simulink model "PCS_average_12_4"  (R2024a)
settings: Solver=FixedStepAuto  StartTime=0.0  StopTime=30.0  RelTol=1e-3
undefined symbols (not defined in the file or in its folder): DiscIntNeverNeededParam, initial, Ion, Lithium
libraries: spsCurrentMeasurementLib x16, spsVoltageMeasurementLib x13, spsControlledVoltageSourceLib x7, spsSeriesRLCBranchLib x5, spsThreePhaseSeriesRLCBranchLib x5, spsGroundLib x2, spsControlledCurrentSourceLib x2, slpidlib x2, SimplusGT x2, spsBatteryLib x1, dspfdesign x1, sps_lib x1
(part 1 of 2)
settings Model: NumberOfSteps=10  Creator=liao  LastModifiedBy=liao

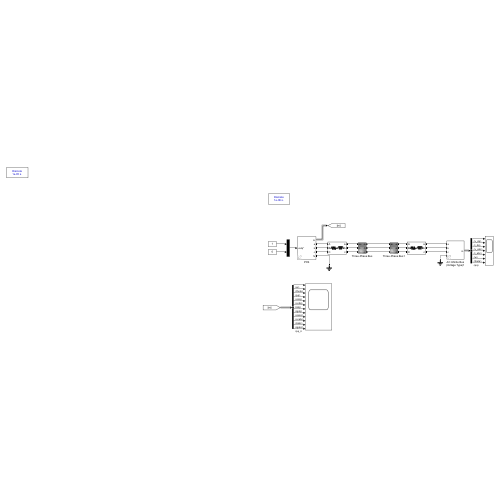
[thumbnail: Simulink's stored preview of the top-level diagram]
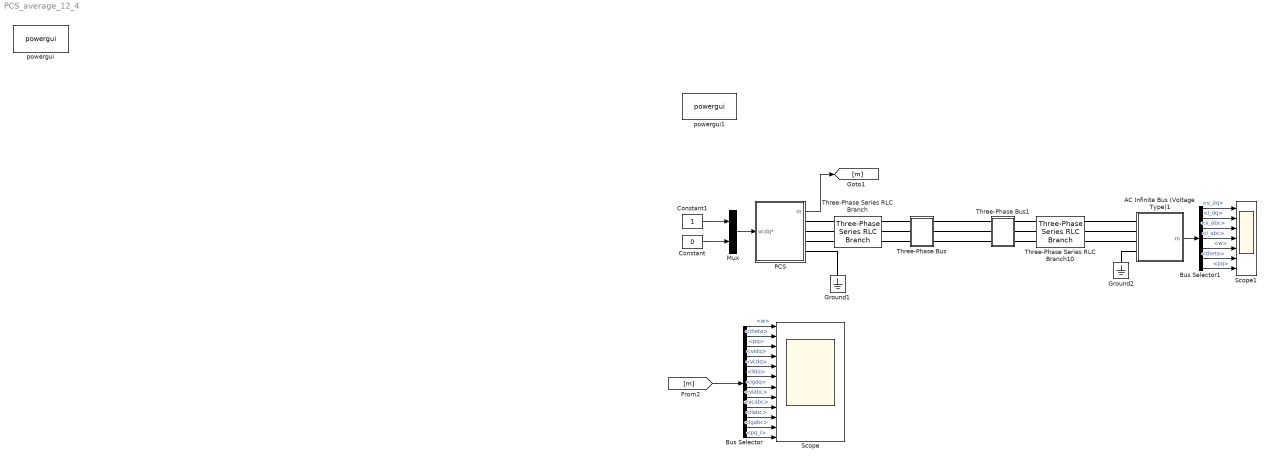
== system PCS_average_12_4 ==
  AC Infinite Bus (Voltage Type)1 : Subsystem  AncestorBlock=|  mask{Ts=1/10e3, Sbase=1, Vbase=1, Wbase=100*pi, vd=1, vq=0, theta0=0, w=100*pi, R=1e-30}
      | SimplusGT/AC Infinite Bus
      | (Voltage Type)
      mask prompts: Ts "Ts (s), samping period"; Sbase "Sbase (VA), power base"; Vbase "Vbase (V), voltage base"; Wbase "Wbase (rad/s), frequency base"; vd "vd (pu), d-axis voltage"; vq "vq (pu), q-axis voltage"; theta0 "theta0 (rad), initial angle"; w "w (rad/s), frequency"; R "R (Ohm), resistance"
      settings: LibrarySourceBlock=|
      | SimplusGT/AC Infinite Bus
      | (Voltage Type)
  Bus Selector : BusSelector  OutputSignals=w,theta,pq,vidq,vcdq,ildq,igdq,viabc,vcabc,ilabc,igabc,pq_i
  Bus Selector1 : BusSelector  OutputSignals=v_dq,i_dq,v_abc,i_abc,w,theta,pq
  Constant : Constant  Value=0
  Constant1 : Constant
  Ground1 : spsGroundLib/Ground  LConnTagsString=a
  Ground2 : spsGroundLib/Ground  LConnTagsString=a
  Mux : Mux  Inputs=2
  PCS : Subsystem  AncestorBlock=|  mask{Ts=1/10e3, Sbase=1, Vbase=1, Wbase=100*pi, w_i=1000*2*pi, w_v=250*2*pi, w_droop=10*2*pi, m=0.08, Lf=0.05, Cf=0.02, Lc=1e-30, Vbase_dc=1, Sbase_dc=1, L_dc=0.000125, C_dc=0.224, Bat_Cap=0.1, SOC_i=100}
      | SimplusGT/Grid-Forming Inverter
      | (Simulink Block)
      mask prompts: Ts "Ts (s), sampling period"; Sbase "Sbase (VA), base power"; Vbase "Vbase (V), base voltage"; Wbase "Wbase (rad/s), base frequency"; w_i "w_i (rad/s), current-loop bandwidth"; w_v "w_v (rad/s), voltage-loop bandwidth"; w_droop "w_droop (rad/s), droop bandwidth"; m "m (pu), frequency droop gain"; Lf "Lf (pu), LCL filter"; Cf "Cf (pu), LCL filter"; Lc "Lc (pu), LCL filter"; Vbase_dc "DC link base voltage"; Sbase_dc "DC link base power"; L_dc "DC link inductance(pu)"; C_dc "DC link super-capacitor(pu)"; Bat_Cap "Battery Capacity(Ah)"; SOC_i "Battery initial State of Charge(%)"
  Scope : Scope  NumInputPorts=12
  Scope1 : Scope  NumInputPorts=7
  Three-Phase Series RLC Branch : spsThreePhaseSeriesRLCBranchLib/Three-Phase Series RLC Branch  LConnTagsString=A|B|C  RConnTagsString=A|B|C  BranchType=RL  Resistance=0.25/5  Inductance=0.25/100/pi  Capacitance=1e-6  Measurements=None
  Three-Phase Series RLC Branch10 : spsThreePhaseSeriesRLCBranchLib/Three-Phase Series RLC Branch  LConnTagsString=A|B|C  RConnTagsString=A|B|C  BranchType=RL  Resistance=0.25/5  Inductance=0.25/100/pi  Capacitance=1e-6  Measurements=None
  Three-Phase Bus : Subsystem  AncestorBlock=SimplusGT/Three-Phase Bus  mask{Vbase=1, Sbase=1}
      settings: LibrarySourceBlock=SimplusGT/Three-Phase Bus
  Three-Phase Bus1 : Subsystem  AncestorBlock=SimplusGT/Three-Phase Bus  mask{Vbase=1, Sbase=1}
      settings: LibrarySourceBlock=SimplusGT/Three-Phase Bus
  powergui : sps_lib/powergui  Priority=1  SimulationMode=Discrete  SampleTime=0.00001  frequency=60  Iterations=50  frequencyindice=0  Pbase=100e6  ErrMax=1e-4  UnitsV=kV  UnitsW=MW  buscounter=0  FunctionMessages=off  echomessages=off  EnableUseOfTLC=off  CurrentSourceSwitches=off  DisableSnubberDevices=off  DisableRonSwitches=off  DisableVfSwitches=off  DisplayEquations=off  AutomaticDiscreteSolvers=off  SolverType=Tustin/Backward Euler (TBE)  Interpol=off  ExternalGateDelay=off  methode=off  Ts=100  x0status=blocks  SPID=on  SwTol=0  HookPort=off  NonlinearTolerance=1e-4  nMaxIteration=100  ContinueOnMaxIteration=off  RestoreLinks=warning  ResistiveCurrentMeasurement=off  Frange=[0:2:500]  Ylog=off  Xlog=on  ShowGrid=off  save=off  variable=ZData  structure=0  ZoomFFT=off  StartTime=0.0  cycles=1  DisplayStyle=1  fundamental=60  FreqAxis=off  MaxFrequency=1000  frequencyindicesteady=1  RmsSteady=1  display=off
  powergui1 : spspowerguiLib/powergui  Priority=1  SimulationMode=Discrete  SampleTime=0.000001  frequency=60  Iterations=50  frequencyindice=0  Pbase=100e6  ErrMax=1e-4  UnitsV=kV  UnitsW=MW  buscounter=0  FunctionMessages=off  echomessages=off  EnableUseOfTLC=off  CurrentSourceSwitches=off  DisableSnubberDevices=off  DisableRonSwitches=off  DisableVfSwitches=off  DisplayEquations=off  AutomaticDiscreteSolvers=off  SolverType=Tustin/Backward Euler (TBE)  Interpol=off  ExternalGateDelay=off  methode=off  Ts=100  x0status=blocks  SPID=on  SwTol=0  HookPort=off  NonlinearTolerance=1e-4  nMaxIteration=100  ContinueOnMaxIteration=off  RestoreLinks=warning  ResistiveCurrentMeasurement=off  Frange=[0:2:500]  Ylog=off  Xlog=on  ShowGrid=off  save=off  variable=ZData  structure=0  ZoomFFT=off  StartTime=0.0  cycles=1  DisplayStyle=1  fundamental=60  FreqAxis=off  MaxFrequency=1000  frequencyindicesteady=1  RmsSteady=1  display=off
  wires:
  Constant/1 -> Mux/2
  Mux/1 -> PCS/1(vcdq*)
  Constant1/1 -> Mux/1
  PCS/1(m) -> [m]
  Bus Selector1/5 -> Scope1/5  "<w>"
  Bus Selector1/1 -> Scope1/1  "<v_dq>"
  Bus Selector1/6 -> Scope1/6  "<theta>"
  Bus Selector1/4 -> Scope1/4  "<i_abc>"
  Bus Selector1/7 -> Scope1/7  "<pq>"
  Bus Selector1/3 -> Scope1/3  "<v_abc>"
  Bus Selector1/2 -> Scope1/2  "<i_dq>"
  AC Infinite Bus (Voltage Type)1/1(m) -> Bus Selector1/1
  [m] -> Bus Selector/1
  Bus Selector/1 -> Scope/1  "<w>"
  Bus Selector/2 -> Scope/2  "<theta>"
  Bus Selector/3 -> Scope/3  "<pq>"
  Bus Selector/4 -> Scope/4  "<vidq>"
  Bus Selector/5 -> Scope/5  "<vcdq>"
  Bus Selector/6 -> Scope/6  "<ildq>"
  Bus Selector/7 -> Scope/7  "<igdq>"
  Bus Selector/8 -> Scope/8  "<viabc>"
  Bus Selector/9 -> Scope/9  "<vcabc>"
  Bus Selector/10 -> Scope/10  "<ilabc>"
  Bus Selector/11 -> Scope/11  "<igabc>"
  Bus Selector/12 -> Scope/12  "<pq_i>"
  connections:
  Three-Phase Bus/RConn1 -- Three-Phase Bus1/LConn1
  Three-Phase Bus/RConn3 -- Three-Phase Bus1/LConn3
  Three-Phase Series RLC Branch10/RConn2 -- AC Infinite Bus (Voltage Type)1/LConn2
  Three-Phase Series RLC Branch10/RConn1 -- AC Infinite Bus (Voltage Type)1/LConn1
  Three-Phase Bus/LConn2 -- Three-Phase Series RLC Branch/RConn2
  Three-Phase Bus/LConn1 -- Three-Phase Series RLC Branch/RConn1
  Three-Phase Bus/LConn3 -- Three-Phase Series RLC Branch/RConn3
  PCS/RConn4 -- Ground1/LConn1
  PCS/RConn1 -- Three-Phase Series RLC Branch/LConn1
  Three-Phase Bus1/RConn2 -- Three-Phase Series RLC Branch10/LConn2
  Three-Phase Bus1/RConn3 -- Three-Phase Series RLC Branch10/LConn3
  Ground2/LConn1 -- AC Infinite Bus (Voltage Type)1/LConn4
  PCS/RConn2 -- Three-Phase Series RLC Branch/LConn2
  Three-Phase Bus1/RConn1 -- Three-Phase Series RLC Branch10/LConn1
  PCS/RConn3 -- Three-Phase Series RLC Branch/LConn3
  Three-Phase Series RLC Branch10/RConn3 -- AC Infinite Bus (Voltage Type)1/LConn3
  Three-Phase Bus/RConn2 -- Three-Phase Bus1/LConn2

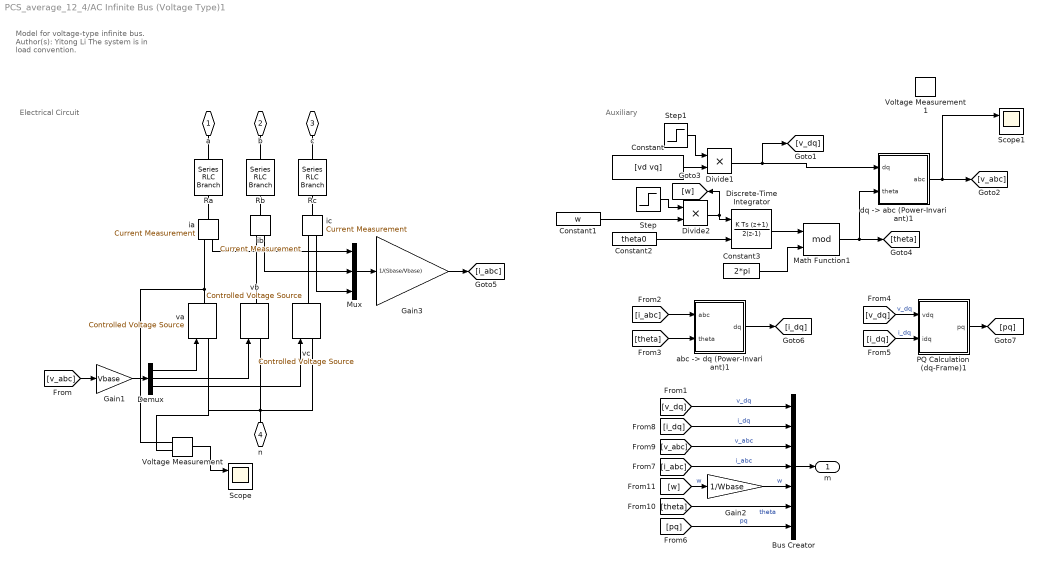
== system PCS_average_12_4/AC Infinite Bus (Voltage Type)1 ==
  note: Auxiliary
  note: Electrical Circuit
  note: Model for voltage-type infinite bus.
      |
      | Author(s): Yitong Li
      |
      | The system is in load convention.
  Bus Creator : BusCreator  Inputs=7
  Constant : Constant  Value=[vd vq]
  Constant1 : Constant  Value=w
  Constant2 : Constant  Value=theta0
  Constant3 : Constant  Value=2*pi
  Demux : Demux  Outputs=3
  Discrete-Time Integrator : DiscreteIntegrator  IntegratorMethod=Integration: Trapezoidal  InitialConditionSource=external  SampleTime=-1  ICPrevOutput=DiscIntNeverNeededParam  ICPrevScaledInput=DiscIntNeverNeededParam
  Divide1 : Product  Inputs=**
  Divide2 : Product  Inputs=**
  Gain1 : Gain  Gain=Vbase
  Gain2 : Gain  Gain=1/Wbase
  Gain3 : Gain  Gain=1/(Sbase/Vbase)
  Math Function1 : Math  Operator=mod  SignedPower=on
  Mux : Mux  Inputs=3
  PQ Calculation (dq-Frame)1 : Subsystem  AncestorBlock=|
      | SimplusGT/PQ Calculation
      | (dq-Frame)
      settings: LibrarySourceBlock=|
      | SimplusGT/PQ Calculation
      | (dq-Frame)
  Ra : spsSeriesRLCBranchLib/Series RLC Branch  LConnTagsString=__new0  RConnTagsString=__new0  BranchType=R  Resistance=R  Inductance=1e-3  SetiL0=off  InitialCurrent=0  Capacitance=1e-6  Setx0=off  InitialVoltage=0  Measurements=None
  Rb : spsSeriesRLCBranchLib/Series RLC Branch  LConnTagsString=__new0  RConnTagsString=__new0  BranchType=R  Resistance=R  Inductance=1e-3  SetiL0=off  InitialCurrent=0  Capacitance=1e-6  Setx0=off  InitialVoltage=0  Measurements=None
  Rc : spsSeriesRLCBranchLib/Series RLC Branch  LConnTagsString=__new0  RConnTagsString=__new0  BranchType=R  Resistance=R  Inductance=1e-3  SetiL0=off  InitialCurrent=0  Capacitance=1e-6  Setx0=off  InitialVoltage=0  Measurements=None
  Scope : Scope  NumInputPorts=2
  Scope1 : Scope  NumInputPorts=2
  Step : Step  Time=15  Before=0.9  After=1.1  SampleTime=0
  Step1 : Step  Time=0.5  Before=1  SampleTime=0
  Voltage Measurement : spsVoltageMeasurementLib/Voltage Measurement  PhasorSimulation=off  OutputType=Complex  PSBequivalent=0
  Voltage Measurement1 : spsVoltageMeasurementLib/Voltage Measurement  PhasorSimulation=off  OutputType=Complex  PSBequivalent=0
  "abc -> dq (Power-Invariant)1" : Subsystem  AncestorBlock=|
      | SimplusGT/abc -> dq
      | (Power-Invariant)
      settings: LibrarySourceBlock=|
      | SimplusGT/abc -> dq
      | (Power-Invariant)
  "dq -> abc (Power-Invariant)1" : Subsystem  AncestorBlock=|
      | SimplusGT/dq -> abc
      | (Power-Invariant)
      settings: LibrarySourceBlock=|
      | SimplusGT/dq -> abc
      | (Power-Invariant)
  ia : spsCurrentMeasurementLib/Current Measurement  PhasorSimulation=off  OutputType=Complex  PSBequivalent=0
  ib : spsCurrentMeasurementLib/Current Measurement  PhasorSimulation=off  OutputType=Complex  PSBequivalent=0
  ic : spsCurrentMeasurementLib/Current Measurement  PhasorSimulation=off  OutputType=Complex  PSBequivalent=0
  va : spsControlledVoltageSourceLib/Controlled Voltage Source  Initialize=on  Source_Type=AC  Amplitude=0  Phase=0  Frequency=0  Measurements=None
  vb : spsControlledVoltageSourceLib/Controlled Voltage Source  Initialize=on  Source_Type=AC  Amplitude=0  Phase=0  Frequency=0  Measurements=None
  vc : spsControlledVoltageSourceLib/Controlled Voltage Source  Initialize=on  Source_Type=AC  Amplitude=0  Phase=0  Frequency=0  Measurements=None
  a : PMIOPort  Side=Left
  b : PMIOPort  Port=2  Side=Left
  c : PMIOPort  Port=3  Side=Left
  n : PMIOPort  Port=4  Side=Left
  m : Outport
  wires:
  [pq] -> Bus Creator/7  "pq"
  PQ Calculation (dq-Frame)1/1(pq) -> [pq]
  [i_dq] -> PQ Calculation (dq-Frame)1/2(idq)  "i_dq"
  [v_dq] -> PQ Calculation (dq-Frame)1/1(vdq)  "v_dq"
  Gain3/1 -> [i_abc]
  Mux/1 -> Gain3/1
  Gain1/1 -> Demux/1
  "abc -> dq (Power-Invariant)1"/1(dq) -> [i_dq]
  [theta] -> "abc -> dq (Power-Invariant)1"/2(theta)
  [i_abc] -> "abc -> dq (Power-Invariant)1"/1(abc)
  ic/1 -> Mux/3
  ib/1 -> Mux/2
  ia/1 -> Mux/1
  [theta] -> Bus Creator/6  "theta"
  Bus Creator/1 -> m/1
  [i_dq] -> Bus Creator/2  "i_dq"
  Gain2/1 -> Bus Creator/5  "w"
  [v_abc] -> Bus Creator/3  "v_abc"
  [w] -> Gain2/1  "w"
  [i_abc] -> Bus Creator/4  "i_abc"
  [v_dq] -> Bus Creator/1  "v_dq"
  Discrete-Time Integrator/1 -> Math Function1/1
  Constant3/1 -> Math Function1/2
  "dq -> abc (Power-Invariant)1"/1(abc) -> Scope1/1, [v_abc]
  Constant1/1 -> Divide2/2
  Constant2/1 -> Discrete-Time Integrator/2
  Math Function1/1 -> [theta], "dq -> abc (Power-Invariant)1"/2(theta)
  Demux/3 -> vc/1
  Demux/2 -> vb/1
  Demux/1 -> va/1
  [v_abc] -> Gain1/1
  Voltage Measurement/1 -> Scope/1
  Step/1 -> Divide2/1
  Divide2/1 -> Discrete-Time Integrator/1, [w]
  Constant/1 -> Divide1/2
  Divide1/1 -> [v_dq], "dq -> abc (Power-Invariant)1"/1(dq)
  Step1/1 -> Divide1/1
  connections:
  Rc/LConn1 -- c/RConn1
  Rc/RConn1 -- ic/LConn1
  Rb/LConn1 -- b/RConn1
  ib/LConn1 -- Rb/RConn1
  Ra/LConn1 -- a/RConn1
  Ra/RConn1 -- ia/LConn1
  ic/RConn1 -- vc/RConn1
  ib/RConn1 -- vb/RConn1
  ia/RConn1 -- Voltage Measurement/LConn1 -- va/RConn1
  vb/LConn1 -- Voltage Measurement/LConn2 -- va/LConn1 -- n/RConn1 -- vc/LConn1

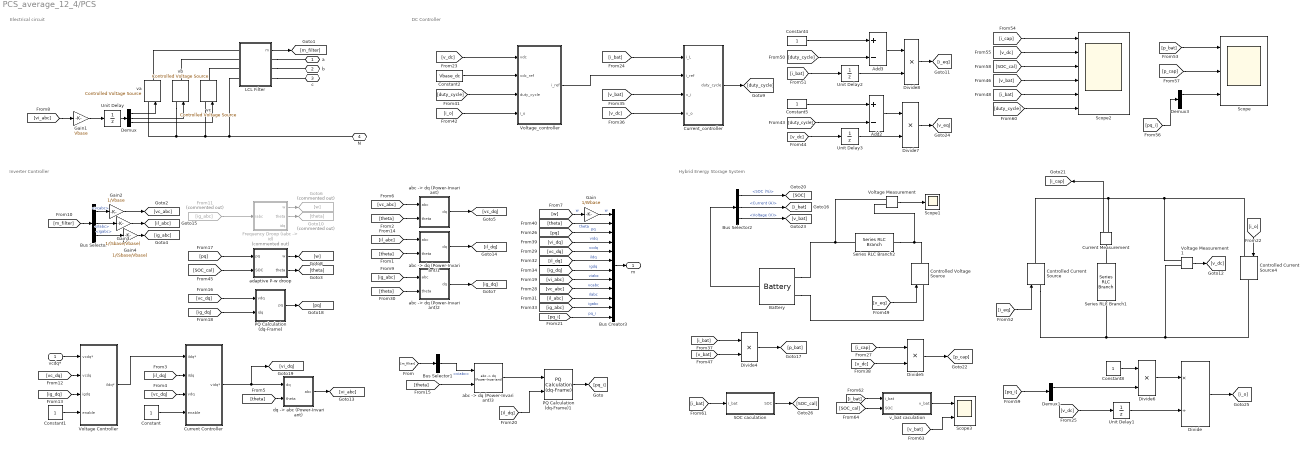
== system PCS_average_12_4/PCS ==
  note: Electrical circuit
  note: Inverter Controller
  note: Hybrid Energy Storage System
  note: DC Controller
  vcdq* : Inport
  Add2 : Sum  Inputs=+-
  Add3 : Sum  Inputs=+-
  Battery : spsBatteryLib/Battery  BatType=Lithium-Ion  ShowTempParam=off  ThermalPreset=no  ShowAgeParam=off  NomV=0.625*Vbase_dc  NomQ=Bat_Cap  SOC=SOC_i  Batt_Tr=30  PresetModel=on  MaxQ=0.1  MinV=0.46875  FullV=0.72749  Dis_rate=0.043478  R=0.0625  Normal_OP=0.090435  expZone="[0.67524    0.004913]"  current=[6.5 16 32.5]  Units=Time  Tci=20  NomT=20  T2=-30  MaxQ2=4.8  FullV2=7.1  Normal_OP2=5.655  expZone2="[6.58           1]"  Rca=0.6  ti=2000  Dp=0  Neq0=0  Tsim=1e6  Ta1=25  Qeol=5.4*0.9  Reol=0.013333*1.2  Char_age=[2.3478, 3]  Dis_age=[2.3478, 10]  N1=1500  N2=10500  N3=1000  N4=1400  Ta2=45  N5=950
  Bus Creator3 : BusCreator  Inputs=12
  Bus Selector : BusSelector  OutputSignals=vcabc,ilabc,igabc
  Bus Selector1 : BusSelector  OutputSignals=viabc
  Bus Selector2 : BusSelector  OutputSignals=SOC (%),Current (A),Voltage (V)
  Constant{,1,4..5,8} (5 alike) : Constant
  Constant2 : Constant  Value=Vbase_dc
  Controlled Current Source : spsControlledCurrentSourceLib/Controlled Current Source  Initialize=on  Source_Type=AC  Amplitude=0  Phase=0  Frequency=0  Measurements=None
  Controlled Current Source4 : spsControlledCurrentSourceLib/Controlled Current Source  Initialize=on  Source_Type=AC  Amplitude=0  Phase=0  Frequency=0  Measurements=None
  Controlled Voltage Source : spsControlledVoltageSourceLib/Controlled Voltage Source  Initialize=on  Source_Type=AC  Amplitude=0  Phase=0  Frequency=0  Measurements=None
  Current Controller : Subsystem  mask{Ts=Ts, Wbase=Wbase, Lf=Lf/Wbase, Kg=0, Kp=w_i*Lf/Wbase, Ki=w_i*w_i/4*Lf/Wbase, xdmax=inf, xqmax=inf, Kcd=0}
      mask prompts: Ts "Sampling Time (s)"; Wbase "Base Angular Frequency (rad/s)"; Lf "Inductance"; Kg "Estimator Gain"; Kp "Proportional Gain"; Ki "Integral Gain"; xdmax "Voltage D Limit"; xqmax "Voltage Q Limit"; Kcd "Cross Decoupling Gain"
  Current Measurement : spsCurrentMeasurementLib/Current Measurement  PhasorSimulation=off  OutputType=Complex  PSBequivalent=0
  Current_controller : Subsystem  mask{w_i=500*2*pi, L=L_dc*Sbase_dc/(Vbase_dc*Vbase_dc), flag_vi_decouple=0, flag_vo_decouple=1}
      mask prompts: w_i "current loop bandwidth"; L "L filter"; flag_vi_decouple "Input voltage decoupling flag"; flag_vo_decouple "Output voltage decoupling flag"
      mask DialogControl ParameterGroupVar Prompt: 参数
  Demux : Demux  Outputs=3
  Demux1 : Demux  Outputs=2
  Demux3 : Demux  Outputs=2
  Divide : Product  Inputs=*/
  Divide{4..8} (5 alike) : Product  Inputs=**
  "Frequency Droop (iabc -> id)" : Subsystem  Commented=on  AncestorBlock=|  mask{Ts=Ts, Sbase=Sbase, Vbase=Vbase, Wbase=Wbase, m=m, w_tau=w_droop, theta0=0, i0=0, w0=1}
      | SimplusGT/Frequency Droop
      | (iabc -> id)
      mask prompts: Ts "Ts (s), samping period"; Sbase "Sbase (VA), base power"; Vbase "Vbase (V), base voltage"; Wbase "Wbase (rad/s), base angular frequency"; m "m (pu), droop gain"; w_tau "w_tau (rad/s), low-pass filter bandwidth"; theta0 "theta0 (rad), initial angle"; i0 "i0 (pu), current setting point"; w0 "w0 (pu), frequency setting point"
  From11 : From  Commented=on  GotoTag=ig_abc
      settings: CloseFcn=tagdialog Close
  Gain : Gain  Gain=1/Wbase
  Gain1 : Gain  Gain=Vbase
  Gain2 : Gain  Gain=1/Vbase
  Gain3 : Gain  Gain=1/(Sbase/Vbase)
  Gain4 : Gain  Gain=1/(Sbase/Vbase)
  Goto10 : Goto  Commented=on  GotoTag=theta
  Goto6 : Goto  Commented=on  GotoTag=w
  LCL Filter : Subsystem  mask{Lf=Lf*(Vbase^2/Sbase)/Wbase, Rf=Lf*(Vbase^2/Sbase)/5, Lc=Lc*(Vbase^2/Sbase)/Wbase, Rc=Lc*(Vbase^2/Sbase)/5, Cf=Cf*(Sbase/Vbase^2)/Wbase, Rd=1e-5*(Vbase^2/Sbase)}
      mask prompts: Lf "Lf (H)"; Rf "Rf (Ohm)"; Lc "Lc (H)"; Rc "Rc (Ohm)"; Cf "Cf (F)"; Rd "Rd (Ohm)"
  PQ Calculation (dq-Frame) : Subsystem  AncestorBlock=|
      | SimplusGT/PQ Calculation
      | (dq-Frame)
  PQ Calculation (dq-Frame)1 : SimplusGT/PQ Calculation (dq-Frame)  SystemSampleTime=-1  VariantActivationTime=update diagram  AllowFlexibleInterface=on  Latency=0  AutoFrameSizeCalculation=off
      settings: SourceProductName=Simplus Grid Tool
  SOC caculation : Subsystem
  Scope : Scope  NumInputPorts=3
  Scope1 : Scope
  Scope2 : Scope  NumInputPorts=6
  Scope3 : Scope  NumInputPorts=2
  Series RLC Branch1 : spsSeriesRLCBranchLib/Series RLC Branch  LConnTagsString=__new0  RConnTagsString=__new0  BranchType=C  Resistance=1  Inductance=1e-3  SetiL0=off  InitialCurrent=0  Capacitance=C_dc*(Vbase_dc*Vbase_dc)/Sbase_dc  Setx0=on  InitialVoltage=Vbase_dc  Measurements=None
  Series RLC Branch2 : spsSeriesRLCBranchLib/Series RLC Branch  LConnTagsString=__new0  RConnTagsString=__new0  BranchType=RL  Resistance=0  Inductance=L_dc*Sbase_dc/(Vbase_dc*Vbase_dc)  SetiL0=on  InitialCurrent=0  Capacitance=1e-6  Setx0=off  InitialVoltage=0  Measurements=None
  Unit Delay : UnitDelay  SampleTime=-1  HasFrameUpgradeWarning=on
  Unit Delay1 : UnitDelay  InitialCondition=Vbase_dc  SampleTime=-1  HasFrameUpgradeWarning=on
  Unit Delay2 : UnitDelay  InitialCondition=Sbase_dc/Vbase_dc  SampleTime=-1  HasFrameUpgradeWarning=on
  Unit Delay3 : UnitDelay  InitialCondition=Vbase_dc  SampleTime=-1  HasFrameUpgradeWarning=on
  Voltage Controller : Subsystem  mask{Ts=Ts, Wbase=Wbase, Cf=Cf/Wbase, Kg=0, Kp=w_v*Cf/Wbase, Ki=w_v*w_v/4*Cf/Wbase*100, xdmax=inf, xqmax=inf, Kcd=0}
      mask prompts: Ts "Sampling Time (s)"; Wbase "Base Angular Frequency (rad/s)"; Cf "Capacitance"; Kg "Estimator Gain"; Kp "Proportional Gain"; Ki "Integral Gain"; xdmax "Current D Limit"; xqmax "Current Q Limit"; Kcd "Cross Decoupling Gain"
  Voltage Measurement : spsVoltageMeasurementLib/Voltage Measurement  PhasorSimulation=off  OutputType=Complex  PSBequivalent=0
  Voltage Measurement1 : spsVoltageMeasurementLib/Voltage Measurement  PhasorSimulation=off  OutputType=Complex  PSBequivalent=0
  Voltage_controller : Subsystem  mask{w_v=50*2*pi, C=C_dc*(Vbase_dc*Vbase_dc)/Sbase_dc, flag_LPF=0, w_LPF=100}
      mask prompts: w_v "voltage loop bandwidth"; C "C filter"; flag_LPF "Use low pass filter"; w_LPF "low pass filter bandwidth"
      mask DialogControl ParameterGroupVar Prompt: 参数
  "abc -> dq (Power-Invariant)" : Subsystem  AncestorBlock=|
      | SimplusGT/abc -> dq
      | (Power-Invariant)
  "abc -> dq (Power-Invariant)1" : Subsystem  AncestorBlock=|
      | SimplusGT/abc -> dq
      | (Power-Invariant)
  "abc -> dq (Power-Invariant)2" : Subsystem  AncestorBlock=|
      | SimplusGT/abc -> dq
      | (Power-Invariant)
  "abc -> dq (Power-Invariant)3" : SimplusGT/abc -> dq (Power-Invariant)  SystemSampleTime=-1  VariantActivationTime=update diagram  AllowFlexibleInterface=on  Latency=0  AutoFrameSizeCalculation=off
      settings: SourceProductName=Simplus Grid Tool
  adaptive P-w droop : Subsystem  mask{Ts=Ts, Sbase=Sbase, Vbase=Vbase, Wbase=Wbase, m=m, w_tau=w_droop, theta0=0, p0=0, w0=1}
      mask prompts: Ts "Ts (s), samping period"; Sbase "Sbase (VA), base power"; Vbase "Vbase (V), base voltage"; Wbase "Wbase (rad/s), base angular frequency"; m "m (pu), droop gain"; w_tau "w_tau (rad/s), low-pass filter bandwidth"; theta0 "theta0 (rad), initial angle"; p0 "p0 (pu), power setting point"; w0 "w0 (pu), frequency setting point"
  "dq -> abc (Power-Invariant)" : Subsystem  AncestorBlock=|
      | SimplusGT/dq -> abc
      | (Power-Invariant)
  v_bat caculation : Subsystem  mask{E=0.67769, A=0.05252, K=0.046158, B=610.6195, R=0.0625}
      mask prompts: E "Nominal voltage"; A "Parameter A"; K "Parameter K"; B "Parameter B"; R "Resistance"
      mask DialogControl ParameterGroupVar Prompt: 参数
  va : spsControlledVoltageSourceLib/Controlled Voltage Source  Initialize=on  Source_Type=AC  Amplitude=0  Phase=0  Frequency=0  Measurements=None
  vb : spsControlledVoltageSourceLib/Controlled Voltage Source  Initialize=on  Source_Type=AC  Amplitude=0  Phase=0  Frequency=0  Measurements=None
  vc : spsControlledVoltageSourceLib/Controlled Voltage Source  Initialize=on  Source_Type=AC  Amplitude=0  Phase=0  Frequency=0  Measurements=None
  a : PMIOPort  Side=Right
  b : PMIOPort  Port=2  Side=Right
  c : PMIOPort  Port=3  Side=Right
  N : PMIOPort  Port=4  Side=Right
  m : Outport
  wires:
  [pq] -> adaptive P-w droop/1(pq)
  adaptive P-w droop/1(w) -> [w]
  adaptive P-w droop/2(theta) -> [theta]
  Gain1/1 -> Unit Delay/1
  [vi_abc] -> Gain1/1
  Gain4/1 -> [ig_abc]
  Gain3/1 -> [il_abc]
  Gain2/1 -> [vc_abc]
  [ig_dq] -> Voltage Controller/3(igdq)
  [vc_dq] -> Voltage Controller/2(vcdq)
  Constant1/1 -> Voltage Controller/4(enable)
  Voltage Controller/1(ildq*) -> Current Controller/1(iIdq*)
  vcdq*/1 -> Voltage Controller/1(vcdq*)
  [ig_abc] -> Bus Creator3/11  "igabc"
  [il_abc] -> Bus Creator3/10  "ilabc"
  [vc_abc] -> Bus Creator3/9  "vcabc"
  [vi_abc] -> Bus Creator3/8  "viabc"
  [ig_dq] -> Bus Creator3/7  "igdq"
  [il_dq] -> Bus Creator3/6  "ildq"
  [vc_dq] -> Bus Creator3/5  "vcdq"
  [vi_dq] -> Bus Creator3/4  "vidq"
  [pq] -> Bus Creator3/3  "pq"
  [theta] -> Bus Creator3/2  "theta"
  Gain/1 -> Bus Creator3/1  "w"
  [w] -> Gain/1  "w"
  Bus Selector/1 -> Gain2/1  "<vcabc>"
  Unit Delay/1 -> Demux/1
  [m_filter] -> Bus Selector/1
  "abc -> dq (Power-Invariant)1"/1(dq) -> [il_dq]
  "abc -> dq (Power-Invariant)2"/1(dq) -> [ig_dq]
  "abc -> dq (Power-Invariant)"/1(dq) -> [vc_dq]
  From11/1 -> "Frequency Droop (iabc -> id)"/1(iabc)
  [il_dq] -> Current Controller/2(iIdq)
  [ig_dq] -> PQ Calculation (dq-Frame)/2(idq)
  PQ Calculation (dq-Frame)/1(pq) -> [pq]
  [vc_dq] -> PQ Calculation (dq-Frame)/1(vdq)
  [theta] -> "dq -> abc (Power-Invariant)"/2(theta)
  Current Controller/1(vidq*) -> "dq -> abc (Power-Invariant)"/1(dq), [vi_dq]
  [vc_dq] -> Current Controller/3(vdq)
  Constant/1 -> Current Controller/4(enable)
  "Frequency Droop (iabc -> id)"/1(w) -> Goto6/1
  "Frequency Droop (iabc -> id)"/2(theta) -> Goto10/1
  Bus Selector/2 -> Gain3/1  "<ilabc>"
  Bus Selector/3 -> Gain4/1  "<igabc>"
  [theta] -> "abc -> dq (Power-Invariant)2"/2(theta)
  [ig_abc] -> "abc -> dq (Power-Invariant)2"/1(abc)
  [il_abc] -> "abc -> dq (Power-Invariant)1"/1(abc)
  [vc_abc] -> "abc -> dq (Power-Invariant)"/1(abc)
  [theta] -> "abc -> dq (Power-Invariant)1"/2(theta)
  [theta] -> "abc -> dq (Power-Invariant)"/2(theta)
  Demux/3 -> vc/1
  Demux/2 -> vb/1
  Demux/1 -> va/1
  LCL Filter/1(m) -> [m_filter]
  Bus Creator3/1 -> m/1
  "dq -> abc (Power-Invariant)"/1(abc) -> [vi_abc]
  [m_filter] -> Bus Selector1/1
  [theta] -> "abc -> dq (Power-Invariant)3"/2
  Bus Selector1/1 -> "abc -> dq (Power-Invariant)3"/1  "<viabc>"
  "abc -> dq (Power-Invariant)3"/1 -> PQ Calculation (dq-Frame)1/1
  [il_dq] -> PQ Calculation (dq-Frame)1/2
  PQ Calculation (dq-Frame)1/1 -> [pq_i]
  [pq_i] -> Bus Creator3/12  "pq_i"
  [v_dc] -> Unit Delay1/1
  [i_eq] -> Controlled Current Source/1
  Bus Selector2/1 -> [SOC]  "<SOC (%)>"
  [i_o] -> Controlled Current Source4/1
  Current Measurement/1 -> [i_cap]
  [v_bat] -> Divide4/2
  [i_bat] -> Divide4/1
  [v_dc] -> Divide5/2
  Unit Delay1/1 -> Divide/2
  Divide6/1 -> Divide/1
  [i_cap] -> Divide5/1
  Divide/1 -> [i_o]
  Constant8/1 -> Divide6/1
  Battery/1 -> Bus Selector2/1
  Voltage Measurement1/1 -> [v_dc]
  [v_eq] -> Controlled Voltage Source/1
  Divide5/1 -> [p_cap]
  Divide4/1 -> [p_bat]
  Constant2/1 -> Voltage_controller/2(vdc_ref)
  [duty_cycle] -> Voltage_controller/3(duty_cycle)
  [v_dc] -> Current_controller/4(v_o)
  [i_bat] -> Current_controller/1(i_L)
  Current_controller/1(duty_cycle) -> [duty_cycle]
  [i_o] -> Voltage_controller/4(i_o)
  [v_bat] -> Current_controller/3(v_i)
  [v_dc] -> Voltage_controller/1(vdc)
  Constant4/1 -> Add3/1
  [v_dc] -> Unit Delay3/1
  [duty_cycle] -> Add3/2
  Divide7/1 -> [v_eq]
  Add3/1 -> Divide8/1
  Divide8/1 -> [i_eq]
  Constant5/1 -> Add2/1
  [duty_cycle] -> Add2/2
  Add2/1 -> Divide7/1
  [v_bat] -> Scope2/4
  [pq_i] -> Demux3/1
  [i_bat] -> Scope2/5
  [v_dc] -> Scope2/2
  [i_cap] -> Scope2/1
  [p_cap] -> Scope/2
  [p_bat] -> Scope/1
  [pq_i] -> Demux1/1
  [SOC_cal] -> Scope2/3
  [i_bat] -> Unit Delay2/1
  Unit Delay2/1 -> Divide8/2
  Unit Delay3/1 -> Divide7/2
  Bus Selector2/2 -> [i_bat]  "<Current (A)>"
  Bus Selector2/3 -> [v_bat]  "<Voltage (V)>"
  [duty_cycle] -> Scope2/6
  Demux3/1 -> Scope/3
  Voltage_controller/1(i_ref) -> Current_controller/2(i_ref)
  [SOC_cal] -> adaptive P-w droop/2(SOC)
  Voltage Measurement/1 -> Scope1/1
  Demux1/1 -> Divide6/2
  [i_bat] -> SOC caculation/1(i_bat)
  SOC caculation/1(SOC) -> [SOC_cal]
  [i_bat] -> v_bat caculation/1(i_bat)
  v_bat caculation/1(v_bat) -> Scope3/1
  [v_bat] -> Scope3/2
  [SOC_cal] -> v_bat caculation/2(SOC)
  connections:
  LCL Filter/LConn3 -- vc/RConn1
  va/LConn1 -- vb/LConn1 -- vc/LConn1 -- LCL Filter/LConn4 -- N/RConn1
  LCL Filter/RConn3 -- c/RConn1
  LCL Filter/RConn2 -- b/RConn1
  LCL Filter/RConn1 -- a/RConn1
  LCL Filter/LConn1 -- va/RConn1
  LCL Filter/LConn2 -- vb/RConn1
  Voltage Measurement1/LConn2 -- Controlled Current Source/LConn1 -- Series RLC Branch1/RConn1 -- Controlled Current Source4/RConn1
  Controlled Current Source/RConn1 -- Controlled Current Source4/LConn1 -- Voltage Measurement1/LConn1 -- Current Measurement/RConn1
  Series RLC Branch2/RConn1 -- Voltage Measurement/LConn2 -- Controlled Voltage Source/RConn1
  Series RLC Branch1/LConn1 -- Current Measurement/LConn1
  Battery/LConn1 -- Voltage Measurement/LConn1 -- Series RLC Branch2/LConn1
  Battery/LConn2 -- Controlled Voltage Source/LConn1

== system PCS_average_12_4/Three-Phase Bus ==
  note: Model for a three-phase bus.
      |
      | Author(s): Yitong Li
      |
      | Notes:
      |
      | It is simply a short-cuirt with current measurement. It is used in the toolbox model for highlighting the position of a bus and making the layout clearer.
  note: Electrical Circuit
  Mux : Mux  Inputs=3
  ia : spsCurrentMeasurementLib/Current Measurement  PhasorSimulation=off  OutputType=Complex  PSBequivalent=0
  ib : spsCurrentMeasurementLib/Current Measurement  PhasorSimulation=off  OutputType=Complex  PSBequivalent=0
  ic : spsCurrentMeasurementLib/Current Measurement  PhasorSimulation=off  OutputType=Complex  PSBequivalent=0
  a+ : PMIOPort  Side=Left
  -a : PMIOPort  Port=2  Side=Right
  b+ : PMIOPort  Port=3  Side=Left
  -b : PMIOPort  Port=4  Side=Right
  c+ : PMIOPort  Port=5  Side=Left
  -c : PMIOPort  Port=6  Side=Right
  wires:
  ic/1 -> Mux/3
  ib/1 -> Mux/2
  ia/1 -> Mux/1
  Mux/1 -> [iabc]
  connections:
  ia/RConn1 -- -a/RConn1
  ia/LConn1 -- a+/RConn1
  ic/LConn1 -- c+/RConn1
  ib/RConn1 -- -b/RConn1
  ib/LConn1 -- b+/RConn1
  ic/RConn1 -- -c/RConn1

== system PCS_average_12_4/Three-Phase Bus1 ==
  note: Model for a three-phase bus.
      |
      | Author(s): Yitong Li
      |
      | Notes:
      |
      | It is simply a short-cuirt with current measurement. It is used in the toolbox model for highlighting the position of a bus and making the layout clearer.
  note: Electrical Circuit
  Mux : Mux  Inputs=3
  ia : spsCurrentMeasurementLib/Current Measurement  PhasorSimulation=off  OutputType=Complex  PSBequivalent=0
  ib : spsCurrentMeasurementLib/Current Measurement  PhasorSimulation=off  OutputType=Complex  PSBequivalent=0
  ic : spsCurrentMeasurementLib/Current Measurement  PhasorSimulation=off  OutputType=Complex  PSBequivalent=0
  a+ : PMIOPort  Side=Left
  -a : PMIOPort  Port=2  Side=Right
  b+ : PMIOPort  Port=3  Side=Left
  -b : PMIOPort  Port=4  Side=Right
  c+ : PMIOPort  Port=5  Side=Left
  -c : PMIOPort  Port=6  Side=Right
  wires:
  ic/1 -> Mux/3
  ib/1 -> Mux/2
  ia/1 -> Mux/1
  Mux/1 -> [iabc]
  connections:
  ia/RConn1 -- -a/RConn1
  ia/LConn1 -- a+/RConn1
  ic/LConn1 -- c+/RConn1
  ib/RConn1 -- -b/RConn1
  ib/LConn1 -- b+/RConn1
  ic/RConn1 -- -c/RConn1

== system PCS_average_12_4/AC Infinite Bus (Voltage Type)1/PQ Calculation (dq-Frame)1 ==
  note: Power calculation.
      |
      | Author(s): Yitong Li
      |
      | Notes:
      |
      | The calculation is done in dq frame.
  vdq : Inport
  idq : Inport  Port=2
  Mux : Mux  Inputs=2
  Mux1 : Mux  Inputs=2
  P = vd*id+vq*iq : Fcn  Expr=u[1]*u[3]+u[2]*u[4]
  Q = -vd*iq+vq*id : Fcn  Expr=-u[1]*u[4]+u[2]*u[3]
  pq : Outport
  wires:
  Mux/1 -> pq/1
  P = vd*id+vq*iq/1 -> Mux/1
  vdq/1 -> Mux1/1
  idq/1 -> Mux1/2
  Mux1/1 -> P = vd*id+vq*iq/1, Q = -vd*iq+vq*id/1
  Q = -vd*iq+vq*id/1 -> Mux/2

== system PCS_average_12_4/AC Infinite Bus (Voltage Type)1/abc -> dq (Power-Invariant)1 ==
  note: Frame transformation from abc to dq.
      |
      | Author(s): Yitong Li
      |
      | Notes:
      |
      | The transformation is power-invariant.
      |
      | theta is the angle that d axis leads a axis.
      |
      | q axis leads d axis by 90 degrees.
  abc : Inport
  theta : Inport  Port=2
  ->d : Fcn  Expr=cos(u(4))*u(1) + cos(u(4)-2/3*pi)*u(2) + cos(u(4)-4/3*pi)*u(3)
  ->q : Fcn  Expr=-sin(u(4))*u(1) - sin(u(4)-2/3*pi)*u(2) - sin(u(4)-4/3*pi)*u(3)
  Gain : Gain  Gain=sqrt(2/3)
  Mux5 : Mux  Inputs=2
  Mux6 : Mux  Inputs=2
  dq : Outport
  wires:
  abc/1 -> Gain/1
  ->d/1 -> Mux6/1
  Gain/1 -> Mux5/1
  theta/1 -> Mux5/2
  ->q/1 -> Mux6/2
  Mux6/1 -> dq/1
  Mux5/1 -> ->d/1, ->q/1

== system PCS_average_12_4/AC Infinite Bus (Voltage Type)1/dq -> abc (Power-Invariant)1 ==
  note: Frame transformation from dq to abc.
      |
      | Author(s): Yitong Li
      |
      | Notes:
      |
      | The transformation is power-invariant.
      |
      | theta is the angle that dq axis leads alpha/beta axis, specifically, d axis leads alpha axis.
  dq : Inport
  theta : Inport  Port=2
  ->a : Fcn  Expr=cos(u(3))*u(1) - sin(u(3))*u(2)
  ->b : Fcn  Expr=cos(u(3)-2/3*pi)*u(1) - sin(u(3)-2/3*pi)*u(2)
  ->c : Fcn  Expr=cos(u(3)-4/3*pi)*u(1) - sin(u(3)-4/3*pi)*u(2)
  Gain : Gain  Gain=sqrt(2/3)
  Mux5 : Mux  Inputs=2
  Mux6 : Mux  Inputs=3
  abc : Outport
  wires:
  ->b/1 -> Mux6/2
  ->a/1 -> Mux6/1
  Gain/1 -> Mux5/1
  dq/1 -> Gain/1
  ->c/1 -> Mux6/3
  Mux6/1 -> abc/1
  Mux5/1 -> ->b/1, ->a/1, ->c/1
  theta/1 -> Mux5/2

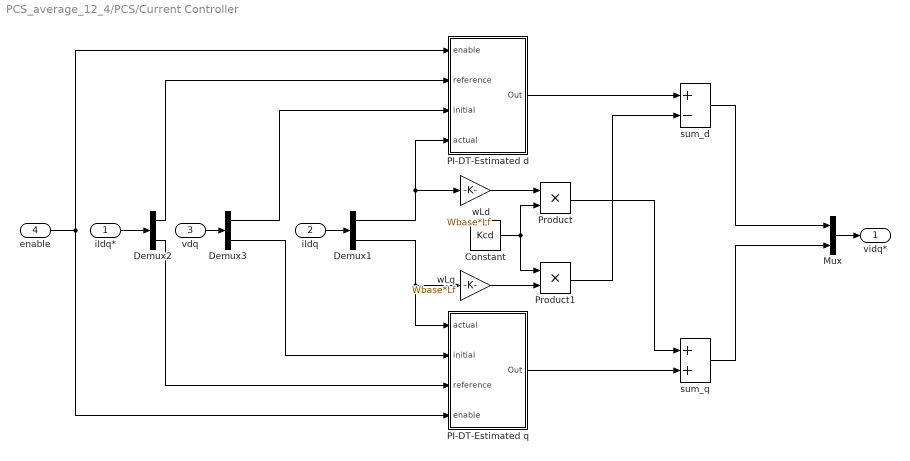
== system PCS_average_12_4/PCS/Current Controller ==
  iIdq* : Inport
  iIdq : Inport  Port=2
  vdq : Inport  Port=3
  enable : Inport  Port=4
  Constant : Constant  Value=Kcd
  Demux1 : Demux  Outputs=2
  Demux2 : Demux  Outputs=2
  Demux3 : Demux  Outputs=2
  Mux : Mux  Inputs=2
  PI-DT-Estimated d : Subsystem  mask{Lf=Lf, Kg=Kg, Kp=Kp, Ki=Ki, xmax=xdmax, xmin=-xdmax, Ts=Ts}
      mask prompts: Lf "Inductance"; Kg "Estimator Gain"; Kp "Proportional Gain"; Ki "Integral Gain"; xmax "Upper Limit"; xmin "Lower Limit"; Ts "Sampling Time"
  PI-DT-Estimated q : Subsystem  mask{Lf=Lf, Kg=Kg, Kp=Kp, Ki=Ki, xmax=xqmax, xmin=-xqmax, Ts=Ts}
      mask prompts: Lf "Inductance"; Kg "Estimator Gain"; Kp "Proportional Gain"; Ki "Integral Gain"; xmax "Upper Limit"; xmin "Lower Limit"; Ts "Sampling Time"
  Product : Product
  Product1 : Product
  sum_d : Sum  Inputs=+-
  sum_q : Sum
  wLd : Gain  Gain=Wbase*Lf
  wLq : Gain  Gain=Wbase*Lf
  vidq* : Outport
  wires:
  Constant/1 -> Product1/1, Product/2
  Product1/1 -> sum_d/2
  wLq/1 -> Product1/2
  Product/1 -> sum_q/1
  wLd/1 -> Product/1
  enable/1 -> PI-DT-Estimated d/1(enable), PI-DT-Estimated q/4(enable)
  Demux2/2 -> PI-DT-Estimated q/3(reference)
  Demux2/1 -> PI-DT-Estimated d/2(reference)
  iIdq*/1 -> Demux2/1
  Demux3/1 -> PI-DT-Estimated d/3(initial)
  Demux3/2 -> PI-DT-Estimated q/2(initial)
  PI-DT-Estimated q/1(Out) -> sum_q/2
  vdq/1 -> Demux3/1
  PI-DT-Estimated d/1(Out) -> sum_d/1
  Mux/1 -> vidq*/1
  Demux1/2 -> wLq/1, PI-DT-Estimated q/1(actual)
  Demux1/1 -> PI-DT-Estimated d/4(actual), wLd/1
  iIdq/1 -> Demux1/1
  sum_q/1 -> Mux/2
  sum_d/1 -> Mux/1

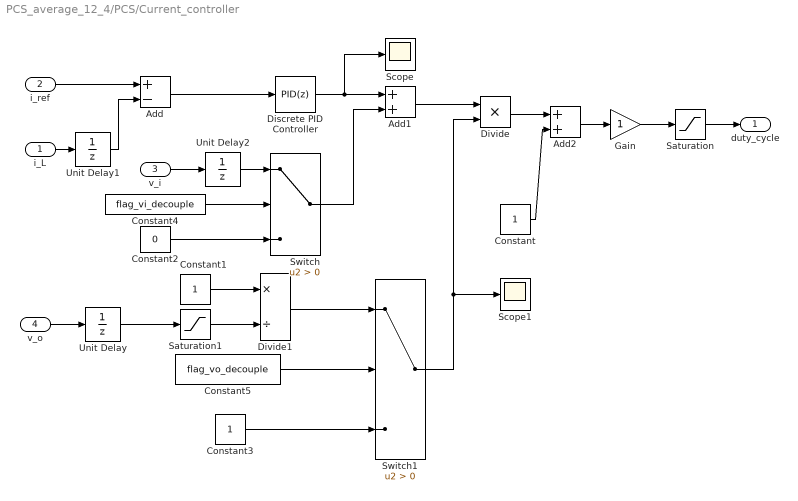
== system PCS_average_12_4/PCS/Current_controller ==
  i_L : Inport
  i_ref : Inport  Port=2
  v_i : Inport  Port=3
  v_o : Inport  Port=4
  Add : Sum  Inputs=+-
  Add1 : Sum
  Add2 : Sum
  Constant : Constant
  Constant1 : Constant
  Constant2 : Constant  Value=0
  Constant3 : Constant
  Constant4 : Constant  Value=flag_vi_decouple
  Constant5 : Constant  Value=flag_vo_decouple
  Discrete PID Controller : slpidlib/PID Controller  Controller=PID  Form=Parallel  TimeDomain=Discrete-time  UseExternalTs=off  SampleTime=-1  IntegratorMethod=Forward Euler  FilterMethod=Forward Euler  ControllerParametersSource=internal  P=w_i*L  I=w_i*w_i*L/4  UseKiTs=off  D=0  UseExternalDerivativeSource=off  N=100  UseFilter=on  TunerSelectOption=Transfer Function Based (PID Tuner App)  InitialConditionSource=internal  InitialConditionForIntegrator=0  InitialConditionForFilter=0  DifferentiatorICPrevScaledInput=0  ExternalReset=none  TrackingMode=off  Kt=1  LimitOutput=off  SatLimitsSource=internal  UpperSaturationLimit=inf  LowerSaturationLimit=-inf  LinearizeAsGain=off  AntiWindupMode=none  Kb=1  LimitIntegrator=off  UpperIntegratorSaturationLimit=inf  LowerIntegratorSaturationLimit=-inf  POutMin=[]  POutMax=[]  IOutMin=[]  IOutMax=[]  DOutMin=[]  DOutMax=[]  NOutMin=[]  NOutMax=[]  SumOutMin=[]  SumOutMax=[]  SaturationOutMin=[]  SaturationOutMax=[]  PParamMin=[]  PParamMax=[]  IParamMin=[]  IParamMax=[]  DParamMin=[]  DParamMax=[]  NParamMin=[]  NParamMax=[]  KbParamMin=[]  KbParamMax=[]  KtParamMin=[]  KtParamMax=[]  KbOutMin=[]  KbOutMax=[]  KtOutMin=[]  KtOutMax=[]  IntegratorOutMin=[]  IntegratorOutMax=[]  FilterOutMin=[]  FilterOutMax=[]  SumI1OutMin=[]  SumI1OutMax=[]  SumI2OutMin=[]  SumI2OutMax=[]  SumI3OutMin=[]  SumI3OutMax=[]  SumI4OutMin=[]  SumI4OutMax=[]  SumDOutMin=[]  SumDOutMax=[]  DifferentiatorOutMin=[]  DifferentiatorOutMax=[]  FilterDiffOutCoefMin=[]  FilterDiffOutCoefMax=[]  ReciprocalOutMin=[]  ReciprocalOutMax=[]  SumDenOutMin=[]  SumDenOutMax=[]  SumNumOutMin=[]  SumNumOutMax=[]  DivideOutMin=[]  DivideOutMax=[]  UdiffTsProdOutMin=[]  UdiffTsProdOutMax=[]  NTsProdOutMin=[]  NTsProdOutMax=[]  UintegralTsProdOutMin=[]  UintegralTsProdOutMax=[]  UngainTsProdOutMin=[]  UngainTsProdOutMax=[]  ClampingZeroOutDataTypeStr=Inherit: Inherit via back propagation  ClampingZeroOutMin=[]  ClampingZeroOutMax=[]  FilterDenConstantOutDataTypeStr=Inherit: Inherit via back propagation  FilterDenConstantOutMin=[]  FilterDenConstantOutMax=[]  PCopyOutDataTypeStr=Inherit: Inherit via back propagation  PCopyOutMin=[]  PCopyOutMax=[]  NCopyOutDataTypeStr=Inherit: Inherit via back propagation  NCopyOutMin=[]  NCopyOutMax=[]  IntegratorContinuousStateAttributes=''  IntegratorStateMustResolveToSignalObject=off  IntegratorRTWStateStorageClass=Auto  FilterContinuousStateAttributes=''  FilterStateMustResolveToSignalObject=off  FilterRTWStateStorageClass=Auto  ParallelPVariant=InternalParameters  IdealPVariant=Disabled  IVariant=InternalParameters  DVariant=InternalParameters  IntegratorVariant=Discrete  SatVariant=Disabled  AWVariant=Passthrough  PCopyVariant=Disabled  TRVariant=Disabled  FdbkBlocksVariant=Forward  IdealPFdbkVariant=Disabled  SatFdbkVariant=Disabled  DerivativeFilterVariant=ForwardEulerFilter  NVariant=InternalParameters  NCopyVariant=Disabled  FilterICVariant=InternalICsFilter  IntegratorICVariant=InternalICs  ExternalResetVariant=Disabled  TRSumVariant=Passthrough  SumFdbkVariant=Disabled  SumVariant=Sum_PID  TsampFilterVariant=InternalTs  TsampNgainVariant=Passthrough  TsampIntegralVariant=Disabled_SignalSpec  ExternalSaturationOutDataTypeStr=Inherit: Same as second input  DerivativeSourceVariant=ErrorSignal
      settings: LibrarySourceBlock=simulink/Discrete/Discrete PID Controller
  Divide : Product  Inputs=**
  Divide1 : Product  Inputs=*/
  Gain : Gain
  Saturation : Saturate  UpperLimit=1  LowerLimit=0
  Saturation1 : Saturate  UpperLimit=inf  LowerLimit=0.1
  Scope : Scope
  Scope1 : Scope
  Switch : Switch  Criteria=u2 > Threshold  SaturateOnIntegerOverflow=off  InputSameDT=off
  Switch1 : Switch  Criteria=u2 > Threshold  SaturateOnIntegerOverflow=off  InputSameDT=off
  Unit Delay : UnitDelay  InitialCondition=Vbase_dc  SampleTime=-1  HasFrameUpgradeWarning=on
  Unit Delay1 : UnitDelay  InitialCondition=0.1  SampleTime=-1  HasFrameUpgradeWarning=on
  Unit Delay2 : UnitDelay  InitialCondition=250  SampleTime=-1  HasFrameUpgradeWarning=on
  duty_cycle : Outport
  wires:
  i_ref/1 -> Add/1
  i_L/1 -> Unit Delay1/1
  Add/1 -> Discrete PID Controller/1
  Discrete PID Controller/1 -> Scope/1, Add1/1
  Add1/1 -> Divide/1
  Constant/1 -> Add2/2
  Add2/1 -> Gain/1
  Saturation/1 -> duty_cycle/1
  Gain/1 -> Saturation/1
  Constant1/1 -> Divide1/1
  Divide/1 -> Add2/1
  v_o/1 -> Unit Delay/1
  Saturation1/1 -> Divide1/2
  Constant4/1 -> Switch/2
  Constant2/1 -> Switch/3
  v_i/1 -> Unit Delay2/1
  Switch/1 -> Add1/2
  Constant3/1 -> Switch1/3
  Constant5/1 -> Switch1/2
  Divide1/1 -> Switch1/1
  Switch1/1 -> Divide/2, Scope1/1
  Unit Delay/1 -> Saturation1/1
  Unit Delay1/1 -> Add/2
  Unit Delay2/1 -> Switch/1

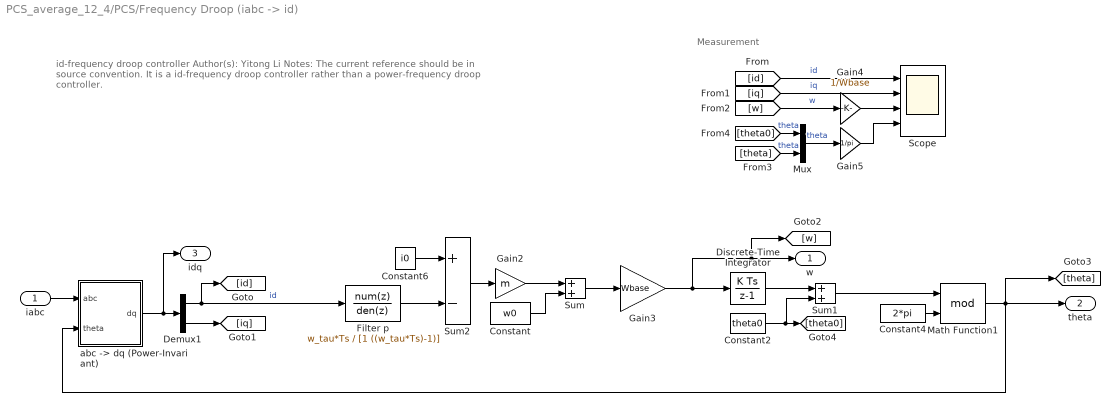
== system PCS_average_12_4/PCS/Frequency Droop (iabc -> id) ==
  note: Measurement
  note: id-frequency droop controller
      |
      | Author(s): Yitong Li
      |
      | Notes:
      |
      | The current reference should be in source convention.
      |
      | It is a id-frequency droop controller rather than a power-frequency droop controller.
  iabc : Inport
  Constant : Constant  Value=w0
  Constant2 : Constant  Value=theta0
  Constant4 : Constant  Value=2*pi
  Constant6 : Constant  Value=i0
  Demux1 : Demux  Outputs=2
  Discrete-Time Integrator : DiscreteIntegrator  SampleTime=Ts  ICPrevOutput=DiscIntNeverNeededParam  ICPrevScaledInput=DiscIntNeverNeededParam
  Filter p : DiscreteTransferFcn  Numerator=w_tau*Ts  Denominator=[1 ((w_tau*Ts)-1)]  SampleTime=Ts
  Gain2 : Gain  Gain=m
  Gain3 : Gain  Gain=Wbase
  Gain4 : Gain  Gain=1/Wbase
  Gain5 : Gain  Gain=1/pi
  Math Function1 : Math  Operator=mod  SignedPower=on
  Mux : Mux  Inputs=2
  Scope : Scope  NumInputPorts=4
  Sum : Sum
  Sum1 : Sum
  Sum2 : Sum  Inputs=+-
  "abc -> dq (Power-Invariant)" : Subsystem  AncestorBlock=|
      | SimplusGT/abc -> dq
      | (Power-Invariant)
  w : Outport
  theta : Outport  Port=2
  idq : Outport  Port=3
  wires:
  Sum1/1 -> Math Function1/1
  Constant2/1 -> Sum1/2, [theta0]
  Math Function1/1 -> "abc -> dq (Power-Invariant)"/2(theta), [theta], theta/1
  Gain2/1 -> Sum/1
  Discrete-Time Integrator/1 -> Sum1/1
  Filter p/1 -> Sum2/2
  Constant/1 -> Sum/2
  "abc -> dq (Power-Invariant)"/1(dq) -> idq/1, Demux1/1
  Constant4/1 -> Math Function1/2
  iabc/1 -> "abc -> dq (Power-Invariant)"/1(abc)
  Constant6/1 -> Sum2/1
  Sum2/1 -> Gain2/1
  Sum/1 -> Gain3/1
  Gain3/1 -> [w], w/1, Discrete-Time Integrator/1
  Demux1/1 -> [id], Filter p/1  "id"
  Gain5/1 -> Scope/4
  [iq] -> Scope/2  "iq"
  [theta0] -> Mux/1  "theta"
  [id] -> Scope/1  "id"
  Mux/1 -> Gain5/1  "theta"
  [theta] -> Mux/2  "theta"
  Demux1/2 -> [iq]
  [w] -> Gain4/1  "w"
  Gain4/1 -> Scope/3

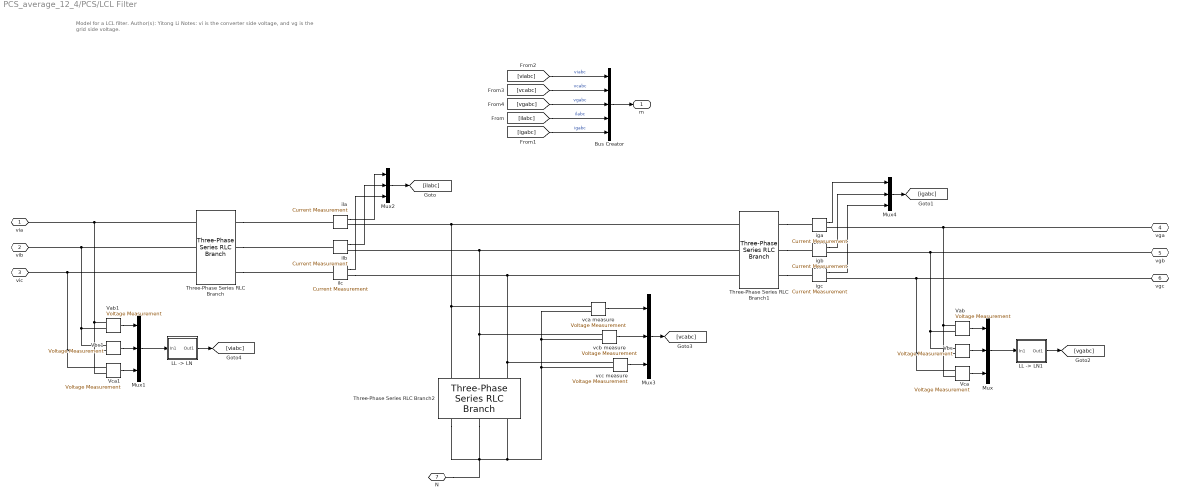
== system PCS_average_12_4/PCS/LCL Filter ==
  note: Model for a LCL filter.
      |
      | Author(s): Yitong Li
      |
      | Notes:
      |
      | vi is the converter side voltage, and vg is the grid side voltage.
  Bus Creator : BusCreator  Inputs=5
  "LL -> LN" : Subsystem  AncestorBlock=SimplusGT/LL -> LN
  "LL -> LN1" : Subsystem  AncestorBlock=|
      | SimplusGT/Grid-Forming Inverter
      | (Simulink Block)/LCL Filter/LL -> LN
  Mux{,1..4} (5 alike) : Mux  Inputs=3
  Three-Phase Series RLC Branch : spsThreePhaseSeriesRLCBranchLib/Three-Phase Series RLC Branch  LConnTagsString=A|B|C  RConnTagsString=A|B|C  BranchType=RL  Resistance=Rf  Inductance=Lf  Capacitance=1e-6  Measurements=None
  Three-Phase Series RLC Branch1 : spsThreePhaseSeriesRLCBranchLib/Three-Phase Series RLC Branch  LConnTagsString=A|B|C  RConnTagsString=A|B|C  BranchType=RL  Resistance=Rc  Inductance=Lc  Capacitance=1e-6  Measurements=None
  Three-Phase Series RLC Branch2 : spsThreePhaseSeriesRLCBranchLib/Three-Phase Series RLC Branch  LConnTagsString=A|B|C  RConnTagsString=A|B|C  BranchType=RC  Resistance=Rd  Inductance=Lc  Capacitance=Cf  Measurements=None
  Vab : spsVoltageMeasurementLib/Voltage Measurement  PhasorSimulation=off  OutputType=Complex  PSBequivalent=0
  Vab1 : spsVoltageMeasurementLib/Voltage Measurement  PhasorSimulation=off  OutputType=Complex  PSBequivalent=0
  Vbc : spsVoltageMeasurementLib/Voltage Measurement  PhasorSimulation=off  OutputType=Complex  PSBequivalent=0
  Vbc1 : spsVoltageMeasurementLib/Voltage Measurement  PhasorSimulation=off  OutputType=Complex  PSBequivalent=0
  Vca : spsVoltageMeasurementLib/Voltage Measurement  PhasorSimulation=off  OutputType=Complex  PSBequivalent=0
  Vca1 : spsVoltageMeasurementLib/Voltage Measurement  PhasorSimulation=off  OutputType=Complex  PSBequivalent=0
  iga : spsCurrentMeasurementLib/Current Measurement  PhasorSimulation=off  OutputType=Complex  PSBequivalent=0
  igb : spsCurrentMeasurementLib/Current Measurement  PhasorSimulation=off  OutputType=Complex  PSBequivalent=0
  igc : spsCurrentMeasurementLib/Current Measurement  PhasorSimulation=off  OutputType=Complex  PSBequivalent=0
  ila : spsCurrentMeasurementLib/Current Measurement  PhasorSimulation=off  OutputType=Complex  PSBequivalent=0
  ilb : spsCurrentMeasurementLib/Current Measurement  PhasorSimulation=off  OutputType=Complex  PSBequivalent=0
  ilc : spsCurrentMeasurementLib/Current Measurement  PhasorSimulation=off  OutputType=Complex  PSBequivalent=0
  vca measure : spsVoltageMeasurementLib/Voltage Measurement  PhasorSimulation=off  OutputType=Complex  PSBequivalent=0
  vcb measure : spsVoltageMeasurementLib/Voltage Measurement  PhasorSimulation=off  OutputType=Complex  PSBequivalent=0
  vcc measure : spsVoltageMeasurementLib/Voltage Measurement  PhasorSimulation=off  OutputType=Complex  PSBequivalent=0
  via : PMIOPort  Side=Left
  vib : PMIOPort  Port=2  Side=Left
  vic : PMIOPort  Port=3  Side=Left
  vga : PMIOPort  Port=4  Side=Right
  vgb : PMIOPort  Port=5  Side=Right
  vgc : PMIOPort  Port=6  Side=Right
  N : PMIOPort  Port=7  Side=Left
  m : Outport
  wires:
  Mux4/1 -> [igabc]
  ilb/1 -> Mux2/2
  ila/1 -> Mux2/1
  igc/1 -> Mux4/3
  vcc measure/1 -> Mux3/3
  Vab/1 -> Mux/1
  Mux/1 -> "LL -> LN1"/1(In1)
  vca measure/1 -> Mux3/1
  vcb measure/1 -> Mux3/2
  igb/1 -> Mux4/2
  iga/1 -> Mux4/1
  Vca/1 -> Mux/3
  ilc/1 -> Mux2/3
  Vbc/1 -> Mux/2
  Mux2/1 -> [ilabc]
  Bus Creator/1 -> m/1
  "LL -> LN1"/1(Out1) -> [vgabc]
  Mux3/1 -> [vcabc]
  Vbc1/1 -> Mux1/2
  Vca1/1 -> Mux1/3
  Mux1/1 -> "LL -> LN"/1(In1)
  Vab1/1 -> Mux1/1
  "LL -> LN"/1(Out1) -> [viabc]
  [viabc] -> Bus Creator/1  "viabc"
  [vcabc] -> Bus Creator/2  "vcabc"
  [vgabc] -> Bus Creator/3  "vgabc"
  [ilabc] -> Bus Creator/4  "ilabc"
  [igabc] -> Bus Creator/5  "igabc"
  connections:
  Three-Phase Series RLC Branch2/RConn1 -- Three-Phase Series RLC Branch2/RConn2 -- N/RConn1 -- Three-Phase Series RLC Branch2/RConn3 -- vcc measure/LConn2 -- vca measure/LConn2 -- vcb measure/LConn2
  Vca/LConn1 -- Vbc/LConn2 -- igc/RConn1 -- vgc/RConn1
  Vca1/LConn1 -- Vbc1/LConn2 -- vic/RConn1 -- Three-Phase Series RLC Branch/LConn3
  Three-Phase Series RLC Branch/LConn2 -- Vbc1/LConn1 -- Vab1/LConn2 -- vib/RConn1
  Vab1/LConn1 -- Vca1/LConn2 -- via/RConn1 -- Three-Phase Series RLC Branch/LConn1
  Three-Phase Series RLC Branch1/LConn3 -- ilc/RConn1 -- Three-Phase Series RLC Branch2/LConn3 -- vcc measure/LConn1
  Three-Phase Series RLC Branch1/RConn2 -- igb/LConn1
  Vbc/LConn1 -- Vab/LConn2 -- igb/RConn1 -- vgb/RConn1
  ilb/RConn1 -- Three-Phase Series RLC Branch1/LConn2 -- vcb measure/LConn1 -- Three-Phase Series RLC Branch2/LConn2
  ila/RConn1 -- Three-Phase Series RLC Branch1/LConn1 -- vca measure/LConn1 -- Three-Phase Series RLC Branch2/LConn1
  Vab/LConn1 -- Vca/LConn2 -- iga/RConn1 -- vga/RConn1
  Three-Phase Series RLC Branch1/RConn1 -- iga/LConn1
  Three-Phase Series RLC Branch1/RConn3 -- igc/LConn1
  Three-Phase Series RLC Branch/RConn1 -- ila/LConn1
  Three-Phase Series RLC Branch/RConn2 -- ilb/LConn1
  Three-Phase Series RLC Branch/RConn3 -- ilc/LConn1

== system PCS_average_12_4/PCS/PQ Calculation (dq-Frame) ==
  note: Power calculation.
      |
      | Author(s): Yitong Li
      |
      | Notes:
      |
      | The calculation is done in dq frame.
  vdq : Inport
  idq : Inport  Port=2
  Mux : Mux  Inputs=2
  Mux1 : Mux  Inputs=2
  P = vd*id+vq*iq : Fcn  Expr=u[1]*u[3]+u[2]*u[4]
  Q = -vd*iq+vq*id : Fcn  Expr=-u[1]*u[4]+u[2]*u[3]
  pq : Outport
  wires:
  Q = -vd*iq+vq*id/1 -> Mux/2
  Mux1/1 -> Q = -vd*iq+vq*id/1, P = vd*id+vq*iq/1
  idq/1 -> Mux1/2
  vdq/1 -> Mux1/1
  P = vd*id+vq*iq/1 -> Mux/1
  Mux/1 -> pq/1

== system PCS_average_12_4/PCS/SOC caculation ==
  i_bat : Inport
  Add : Sum
  Constant3 : Constant  Value=SOC_i/100
  Constant6 : Constant  Value=-Bat_Cap*3600
  Discrete-Time Integrator : DiscreteIntegrator  SampleTime=-1  ICPrevOutput=DiscIntNeverNeededParam  ICPrevScaledInput=DiscIntNeverNeededParam
  Divide1 : Product  Inputs=*/
  SOC : Outport
  wires:
  Constant3/1 -> Add/2
  Discrete-Time Integrator/1 -> Divide1/1
  Constant6/1 -> Divide1/2
  i_bat/1 -> Discrete-Time Integrator/1
  Divide1/1 -> Add/1
  Add/1 -> SOC/1

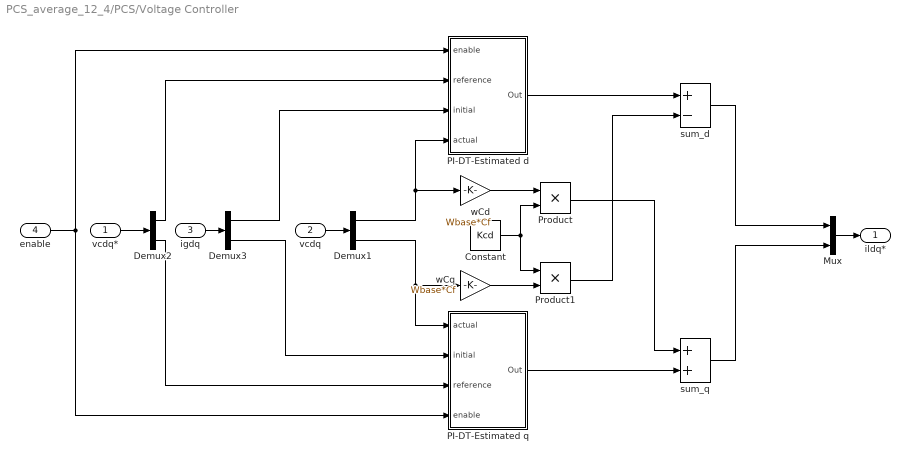
== system PCS_average_12_4/PCS/Voltage Controller ==
  vcdq* : Inport
  vcdq : Inport  Port=2
  igdq : Inport  Port=3
  enable : Inport  Port=4
  Constant : Constant  Value=Kcd
  Demux1 : Demux  Outputs=2
  Demux2 : Demux  Outputs=2
  Demux3 : Demux  Outputs=2
  Mux : Mux  Inputs=2
  PI-DT-Estimated d : Subsystem  mask{Kg=Kg, Kp=Kp, Ki=Ki, xmax=xdmax, xmin=-xdmax, Ts=Ts}
      mask prompts: Kg "Estimator Gain"; Kp "Proportional Gain"; Ki "Integral Gain"; xmax "Upper Limit"; xmin "Lower Limit"; Ts "Sampling Time"
  PI-DT-Estimated q : Subsystem  mask{Kg=Kg, Kp=Kp, Ki=Ki, xmax=xqmax, xmin=-xqmax, Ts=Ts}
      mask prompts: Kg "Estimator Gain"; Kp "Proportional Gain"; Ki "Integral Gain"; xmax "Upper Limit"; xmin "Lower Limit"; Ts "Sampling Time"
  Product : Product
  Product1 : Product
  sum_d : Sum  Inputs=+-
  sum_q : Sum
  wCd : Gain  Gain=Wbase*Cf
  wCq : Gain  Gain=Wbase*Cf
  ildq* : Outport
  wires:
  Constant/1 -> Product1/1, Product/2
  Product1/1 -> sum_d/2
  wCq/1 -> Product1/2
  Product/1 -> sum_q/1
  wCd/1 -> Product/1
  enable/1 -> PI-DT-Estimated d/1(enable), PI-DT-Estimated q/4(enable)
  Demux2/2 -> PI-DT-Estimated q/3(reference)
  Demux2/1 -> PI-DT-Estimated d/2(reference)
  vcdq*/1 -> Demux2/1
  Demux3/1 -> PI-DT-Estimated d/3(initial)
  Demux3/2 -> PI-DT-Estimated q/2(initial)
  PI-DT-Estimated q/1(Out) -> sum_q/2
  igdq/1 -> Demux3/1
  PI-DT-Estimated d/1(Out) -> sum_d/1
  Mux/1 -> ildq*/1
  Demux1/2 -> wCq/1, PI-DT-Estimated q/1(actual)
  Demux1/1 -> PI-DT-Estimated d/4(actual), wCd/1
  vcdq/1 -> Demux1/1
  sum_q/1 -> Mux/2
  sum_d/1 -> Mux/1
